simulink model "RosTest"  (R2020b)
settings: Solver=VariableStepAuto  StartTime=0.0  StopTime=inf  RelTol=1e-3
libraries: robotlib x1
settings Model: Creator=51078  LastModifiedBy=51078
settings DataIOCC: ReturnWorkspaceOutputs=off
settings DebuggingCC: ArithmeticOperatorsInVariantConditions=warning
settings SFSimCC: CustomCodeUndefinedFunction=UseInterfaceOnly

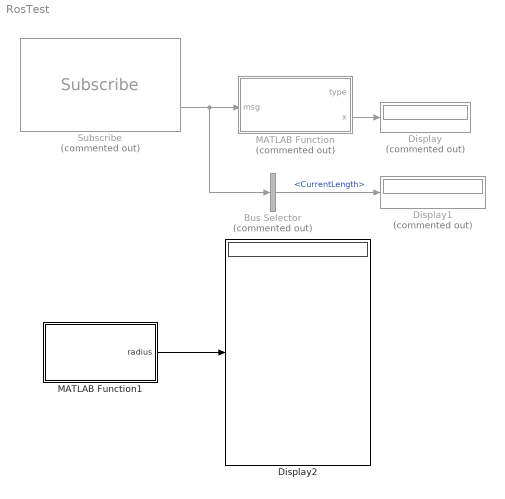
== system RosTest ==
  Bus Selector : BusSelector  Commented=on  OutputSignals=Units_SL_Info.CurrentLength
  Display : Display  Commented=on
  Display1 : Display  Commented=on
  Display2 : Display
  MATLAB Function : MATLAB Function  Commented=on  TreatAsAtomicUnit=on
  MATLAB Function1 : MATLAB Function
  Subscribe : robotlib/Subscribe  Commented=on  topicSource=Select from ROS network  topic=/decision_info  messageType=swarm_msgs/Pipeline  SampleTime=-1  legacyBusStruct=off  messageQueueLength=1
  wires:
  Subscribe/2 -> Bus Selector/1, MATLAB Function/1(msg)
  MATLAB Function/2(x) -> Display/1
  Bus Selector/1 -> Display1/1  "<CurrentLength>"
  MATLAB Function1/1(radius) -> Display2/1

== matlab function RosTest/MATLAB Function1 ==
  data: radius output
function radius   = fcn
coder.extrinsic('csape')
EncirclePoint=[113,1.7;161,-9;211,-5;248,-18;262,-6;260,13;252,27;202,29;132,23;116,16;113,1.7];
EncirclePoint_x=EncirclePoint(:,1);
EncirclePoint_y=EncirclePoint(:,2);
k=length(EncirclePoint_x);
xx=csape(1:k,EncirclePoint_x,'periodic');
yy=csape(1:k,EncirclePoint_y,'periodic');
curve_x=ppval(xx,linspace(1,k,100*k));
curve_y=ppval(yy,linspace(1,k,100*k));

radius=zeros(100*k,2);
for i=1:length(radius(:,1))
    radius(i,1)=curve_x(i);
    radius(i,2)=curve_y(i);
end

== matlab function RosTest/MATLAB Function ==
  data: type output; msg input; x output
function [type,x] = fcn(msg)
type = msg.Pipetype.Data;
x = msg.Units(17).Right.X;
